simulink model "AOO_stateflow"  (R2022a)
settings: Solver=FixedStepAuto  StartTime=0.0  StopTime=0.002  FixedStep=1e-3  RelTol=1e-3  EnableMultiTasking=on
undefined symbols (not defined in the file): D0, D1, D11, D12, D2, D4, D5, D7, D8, D9, PTA0, PTA2, PTB23, PTB9, PTC16, PTC17, PTC3, PTC4, PTD2, PTD3
libraries: frdmk64flib x10
settings Model: SimulationMode=external  ExtModeTrigDuration=5  Creator=22363  LastModifiedBy=22363
settings OptimizationCC: EnhancedBackFolding=on  PassReuseOutputArgsAs=Individual arguments  ZeroExternalMemoryAtStartup=off  ZeroInternalMemoryAtStartup=off  MaxStackSize=64  OptimizeBlockOrder=speed  DifferentSizesBufferReuse=on  OptimizationCustomize=off  EfficientTunableParamExpr=on
settings DebuggingCC: ParameterTunabilityLossMsg=error
settings HardwareCC: ProdBitPerPointer=32  ProdBitPerSizeT=32  ProdBitPerPtrDiffT=32  ProdLargestAtomicInteger=Long  ProdLargestAtomicFloat=Double  ProdWordSize=32  ProdHWDeviceType=ARM Compatible->ARM Cortex
settings SFSimCC: MATLABDynamicMemAlloc=off
settings RTWCC: SystemTargetFile=ert.tlc  HardwareBoard=NXP FRDM-K64F  TLCOptions="-aInlineSetEventsForThisBaseRateFcn=TLC_FALSE -aSuppressMultiTaskScheduler=TLC_FALSE  -aRateBasedStepFcn=0"  TemplateMakefile=ert_default_tmf  Toolchain=GNU Tools for ARM Embedded Processors
settings CodeAppCC: ForceParamTrailComments=on  IgnoreCustomStorageClasses=off  OperatorAnnotations=on  SimulinkDataObjDesc=on  SFDataObjDesc=on  InsertBlockDesc=on
settings ERTTargetCC: ExtMode=on  ExtModeTransport=6  ExtModeMexFile=sendToCommService  ExtModeMexArgs='AOO_stateflow' 0

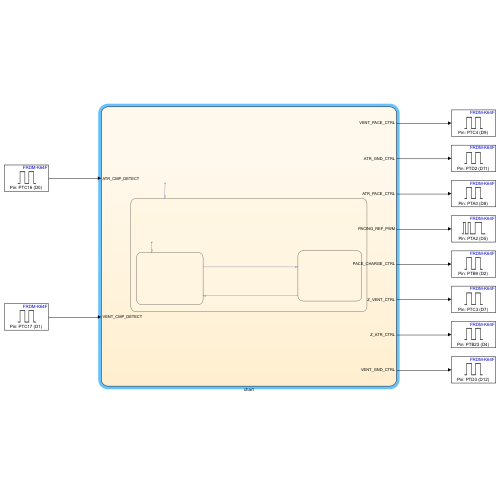
[thumbnail: Simulink's stored preview of the top-level diagram]
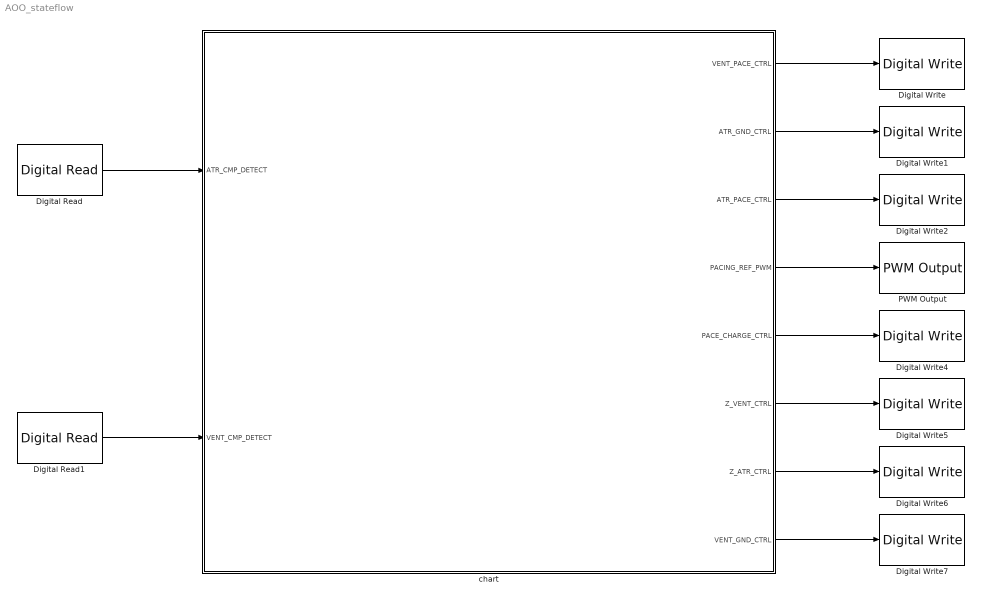
== system AOO_stateflow ==
  Digital Read : frdmk64flib/Digital Read  Whichpin=PTC16 (D0)  SampleTime=-1
  Digital Read1 : frdmk64flib/Digital Read  Whichpin=PTC17 (D1)  SampleTime=-1
  Digital Write : frdmk64flib/Digital Write  Whichpin=PTC4 (D9)
  Digital Write1 : frdmk64flib/Digital Write  Whichpin=PTD2 (D11)
  Digital Write2 : frdmk64flib/Digital Write  Whichpin=PTA0 (D8)
  Digital Write4 : frdmk64flib/Digital Write  Whichpin=PTB9 (D2)
  Digital Write5 : frdmk64flib/Digital Write  Whichpin=PTC3 (D7)
  Digital Write6 : frdmk64flib/Digital Write  Whichpin=PTB23 (D4)
  Digital Write7 : frdmk64flib/Digital Write  Whichpin=PTD3 (D12)
  PWM Output : frdmk64flib/PWM Output  Whichpin=PTA2 (D5)  InitialFrequency=2000  InitialDutyCycle=50
  chart : Stateflow chart  TreatAsAtomicUnit=on
  wires:
  chart/8(VENT_GND_CTRL) -> Digital Write7/1
  chart/7(Z_ATR_CTRL) -> Digital Write6/1
  chart/6(Z_VENT_CTRL) -> Digital Write5/1
  chart/5(PACE_CHARGE_CTRL) -> Digital Write4/1
  chart/4(PACING_REF_PWM) -> PWM Output/1
  chart/3(ATR_PACE_CTRL) -> Digital Write2/1
  chart/2(ATR_GND_CTRL) -> Digital Write1/1
  chart/1(VENT_PACE_CTRL) -> Digital Write/1
  Digital Read/1 -> chart/1(ATR_CMP_DETECT)
  Digital Read1/1 -> chart/2(VENT_CMP_DETECT)

== stateflow chart AOO_stateflow/chart ==
  state AOO_Mode
    entry:
    ATR_PACE_CTRL = 0;
    VENT_PACE_CTRL = 0;
    PACE_CHARGE_CTRL = 0;
    Z_VENT_CTRL = 0;
    Z_ATR_CTRL = 0;
    PACING_REF_PWM = ATR_PULSE_WIDTH/1000;
    state SendPulse
      entry:
      PACE_CHARGE_CTRL = 0;
      ATR_PACE_CTRL = 1;
      ATR_GND_CTRL = 0;
      PACE_CHARGE_CTRL = 1;
      %
      VENT_PACE_CTRL = 0;
      VENT_GND_CTRL = 0;
    state ReadyPulse
      entry:
      PACE_CHARGE_CTRL = 1;
      ATR_PACE_CTRL = 0;
      ATR_GND_CTRL = 1;
      PACE_CHARGE_CTRL = 0;
      %
      VENT_PACE_CTRL = 0;
      VENT_GND_CTRL = 0;
    (default) -> ReadyPulse
    ReadyPulse -> SendPulse : after(LRI - ATR_PULSE_WIDTH,msec)
    SendPulse -> ReadyPulse : after(ATR_PULSE_WIDTH,msec)
  (default) -> AOO_Mode
  data: LRI constant double =1000; VENT_PACE_CTRL output; ATR_GND_CTRL output; ATR_PACE_CTRL output; PACING_REF_PWM output; PACE_CHARGE_CTRL output; Z_VENT_CTRL output; Z_ATR_CTRL output; VENT_GND_CTRL output; ATR_CMP_DETECT input; VENT_CMP_DETECT input; ATR_PULSE_WIDTH constant double =0.4; VENT_PULSE_WIDTH constant double =0.4
